simulink model "bianpinx1"  (R2015b)
settings: Solver=ode23t  StartTime=0.0  StopTime=0.4  RelTol=1e-3
libraries: powerlib x22, powerlib_extras x2
settings Model: Creator=Administrator  LastModifiedBy=Administrator
settings DataIOCC: SaveFormat=Array  SignalLoggingSaveFormat=ModelDataLogs
settings OptimizationCC: BooleanDataType=off  InitFltsAndDblsToZero=on
settings DebuggingCC: SaveWithParameterizedLinksMsg=none  UnderspecifiedInitializationDetection=Classic  MergeDetectMultiDrivingBlocksExec=none  SignalResolutionControl=TryResolveAllWithWarning  MaxConsecutiveZCsMsg=none  MultiTaskDSMMsg=warning  MultiTaskCondExecSysMsg=none  FcnCallInpInsideContextMsg=UseLocalSettings
settings HardwareCC: ProdBitPerPointer=32  ProdLargestAtomicFloat=None  ProdIntDivRoundTo=Undefined  ProdEndianess=Unspecified  ProdWordSize=32  ProdHWDeviceType=32-bit Generic  TargetUnknown=on
settings GRTTargetCC: TargetFcnLib=ansi_tfl_tmw.mat  CombineOutputUpdateFcns=off  GRTInterface=on
settings ConfigComp: CovModelRefEnable=Off

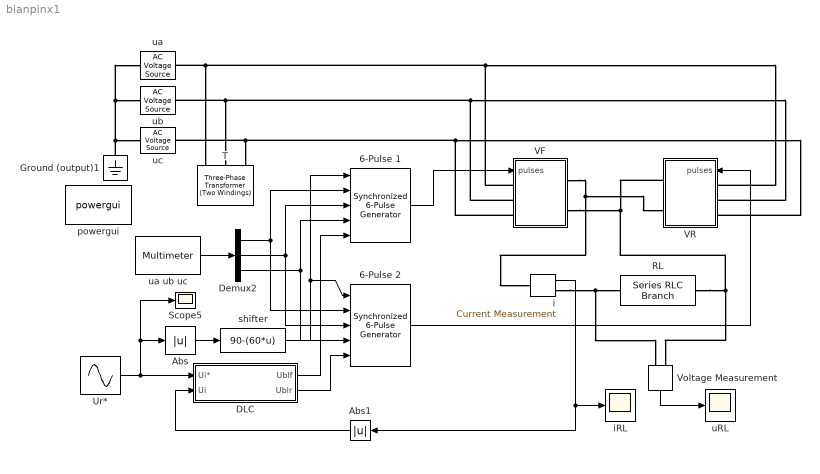
== system bianpinx1 ==
  "6-Pulse 1 " : powerlib_extras/Control  Blocks/Synchronized 6-Pulse Generator  freq=50  pwidth=10  Double_Pulse=on
  6-Pulse 2 : powerlib_extras/Control  Blocks/Synchronized 6-Pulse Generator  freq=50  pwidth=10  Double_Pulse=on
  Abs : Abs  SaturateOnIntegerOverflow=on
  Abs1 : Abs  SaturateOnIntegerOverflow=on
  DLC : Subsystem
  Demux2 : Demux  Outputs=3
  Ground (output)1 : powerlib/Elements/Ground  LConnTagsString=a
  RL : powerlib/Elements/Series RLC Branch  LConnTagsString=__new0  RConnTagsString=__new0  BranchType=RL  Resistance=1  Inductance=0.01  SetiL0=off  InitialCurrent=0  Capacitance=[]  Setx0=off  InitialVoltage=0  Measurements=Branch voltage and current
  Scope5 : Scope
  T : powerlib/Elements/Three-Phase Transformer (Two Windings)  Winding1Connection=Y  Winding2Connection=Y  CoreType=Three single-phase transformers  SetSaturation=off  Hysteresis=off  DataFile='basic_model'  SetInitialFlux=off  Measurements=Winding voltages  UNITS=pu  NominalPower=[ 250e6 , 50 ]  Winding1=[380, 0.002 , 0.08 ]  Winding2=[12.25 , 0.002 , 0.08 ]  Rm=500  Lm=500  L0=0.5  Saturation="[ 0,0  ;  0.005,1.2  ;  1.0,1.4 ]"  InitialFluxes=[ 0.8 , -0.8 , 0.7 ]  MoreParameters=off  BreakLoop=off  DataType=off  TransfoNumber=0
  Ur* : Sin  Frequency=2*pi*10  SampleTime=0
  VF : Subsystem  AncestorBlock=|  mask(Six-pulse thyristor bridge){Ron=0.01, Lon=10e-6, Rs=1e3, Cs=1e-6}
      | powerlib_extras/Three-Phase
      | Library/6 - pulse
      |  thyristor bridge
      mask prompts: Ron "Thyristor on-state resitance (Ohms) :"; Lon "Thyristor on-state inductance (H) :"; Rs "Snubber resistance (Ohms) :"; Cs "Snubber capacitance (F) :"
      mask help:
      | This block implements a six-pulses thyristor bridge rectifier with RC snubbers. Set the snubber resistance to Inf to remove all the thyristors snubbers. This block uses six Simplified Thyristors from the powerlib/Power Electronics library.
      | Input four (labeled 'pulses') of the block is a Simulink vector of length six that  controls the thyristors gates. Use the 'Look Under Mask' in the Edit menu  to see how the control vector operates the six thyrsistors.
      mask init:
      | power_initmask();
      settings: OpenFcn=power_openblockproxy()
      mask Display: plot(0,0,100,100,[50,50,35,50,65,50],[30,40,40,60,40,40],[35,65],[60,60],[50,50],[60,70],[45,40],[60,65],[35,40],[65,65])
  VR : Subsystem  AncestorBlock=|  mask(Six-pulse thyristor bridge){Ron=0.01, Lon=10e-6, Rs=1e3, Cs=1e-6}
      | powerlib_extras/Three-Phase
      | Library/6 - pulse
      |  thyristor bridge
      mask prompts: Ron "Thyristor on-state resitance (Ohms) :"; Lon "Thyristor on-state inductance (H) :"; Rs "Snubber resistance (Ohms) :"; Cs "Snubber capacitance (F) :"
      mask help:
      | This block implements a six-pulses thyristor bridge rectifier with RC snubbers. Set the snubber resistance to Inf to remove all the thyristors snubbers. This block uses six Simplified Thyristors from the powerlib/Power Electronics library.
      | Input four (labeled 'pulses') of the block is a Simulink vector of length six that  controls the thyristors gates. Use the 'Look Under Mask' in the Edit menu  to see how the control vector operates the six thyrsistors.
      mask init:
      | power_initmask();
      settings: OpenFcn=power_openblockproxy()
      mask Display: plot(0,0,100,100,[50,50,35,50,65,50],[30,40,40,60,40,40],[35,65],[60,60],[50,50],[60,70],[45,40],[60,65],[35,40],[65,65])
  Voltage Measurement : powerlib/Measurements/Voltage Measurement  PhasorSimulation=off  OutputType=Complex  PSBequivalent=0
  i : powerlib/Measurements/Current Measurement  PhasorSimulation=off  OutputType=Magnitude  PSBequivalent=0
  iRL : Scope
  powergui : powerlib/powergui  Priority=1  SimulationMode=Continuous  SolverType=Tustin/Backward Euler (TBE)  SampleTime=50e-6  frequency=60  SPID=off  DisableSnubberDevices=off  DisableRonSwitches=off  DisableVfSwitches=off  SwTol=0  DisplayEquations=off  Interpol=off  ExternalGateDelay=off  methode=off  Ts=10  FunctionMessages=off  echomessages=off  HookPort=off  EnableUseOfTLC=off  x0status=blocks  frequencyindice=50  Pbase=100e6  ErrMax=1e-4  Iterations=50  UnitsV=kV  UnitsW=MW  buscounter=0  RestoreLinks=warning  ResistiveCurrentMeasurement=off  Frange=[0:2:500]  Ylog=off  Xlog=on  ShowGrid=off  save=off  variable=ZData  structure=0  ZoomFFT=off  StartTime=0.0  cycles=1  DisplayStyle=1  fundamental=60  FreqAxis=off  MaxFrequency=1000  frequencyindicesteady=1  RmsSteady=1  display=off
  shifter : Fcn  Expr=90-(60*u)
  uRL : Scope
  ua : powerlib/Electrical Sources/AC Voltage Source  Amplitude=311  Phase=0  Frequency=50  SampleTime=0  Measurements=Voltage  BusType=swing  Pref=10e3  Qref=0  Qmin=-inf  Qmax=+inf
  ua ub uc : powerlib/Measurements/Multimeter  PhasorSimulation=off  OutputType=Magnitude  sel=[5 6 7]  L=11  Gain=[1 1 1]  yselected={'Uan_w2: T','Ubn_w2: T','Ucn_w2: T'};  PSBOutputType=1  PSBequivalent=0  AxesSetting=[0,0.1,-100,100]  Display=0  SavedBlockNames=-11
  ub : powerlib/Electrical Sources/AC Voltage Source  Amplitude=311  Phase=-120  Frequency=50  SampleTime=0  Measurements=Voltage  BusType=swing  Pref=10e3  Qref=0  Qmin=-inf  Qmax=+inf
  uc : powerlib/Electrical Sources/AC Voltage Source  Amplitude=311  Phase=-240  Frequency=50  SampleTime=0  Measurements=Voltage  BusType=swing  Pref=10e3  Qref=0  Qmin=-inf  Qmax=+inf
  wires:
  6-Pulse 2/1 -> VR/1(pulses)
  Ur*/1 -> Abs/1, Scope5/1, DLC/1(Ui*)
  DLC/1(Ublf) -> "6-Pulse 1 "/5
  DLC/2(Ublr) -> 6-Pulse 2/5
  Abs/1 -> shifter/1
  shifter/1 -> "6-Pulse 1 "/1, 6-Pulse 2/1
  Demux2/1 -> "6-Pulse 1 "/2, 6-Pulse 2/2
  Demux2/2 -> "6-Pulse 1 "/3, 6-Pulse 2/3
  Demux2/3 -> "6-Pulse 1 "/4, 6-Pulse 2/4
  Abs1/1 -> DLC/2(Ui)
  ua ub uc/1 -> Demux2/1
  i/1 -> Abs1/1, iRL/1
  Voltage Measurement/1 -> uRL/1
  "6-Pulse 1 "/1 -> VF/1(pulses)
  connections:
  Ground (output)1/LConn1 -- ua/LConn1 -- ub/LConn1 -- uc/LConn1
  i/RConn1 -- RL/LConn1 -- Voltage Measurement/LConn1
  RL/RConn1 -- VF/RConn2 -- VR/RConn1 -- Voltage Measurement/LConn2
  VF/RConn1 -- VR/RConn2 -- i/LConn1
  VF/LConn1 -- VR/LConn1 -- ua/RConn1 -- T/LConn1
  VF/LConn2 -- VR/LConn2 -- ub/RConn1 -- T/LConn2
  VF/LConn3 -- VR/LConn3 -- uc/RConn1 -- T/LConn3

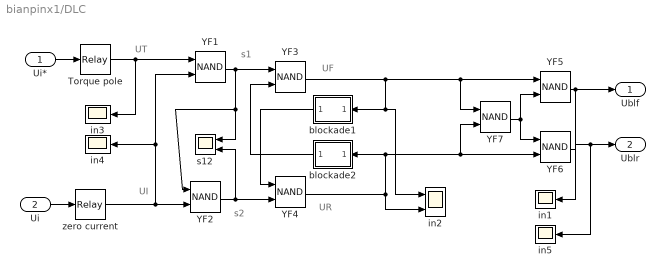
== system bianpinx1/DLC ==
  note: s1
  note: s2
  note: UT
  note: UI
  note: UF
  note: UR
  Ui* : Inport
  Ui : Inport  Port=2
  Torque pole : Relay  OnSwitchValue=0.001  OffSwitchValue=-0.001
  YF{1..7} (7 alike) : Logic  Operator=NAND
  blockade1 : Subsystem
  blockade2 : Subsystem
  in{1,3..5} (4 alike) : Scope
  in2 : Scope  NumInputPorts=2
  s12 : Scope  NumInputPorts=2
  "zero current  " : Relay  OnSwitchValue=0.5  OffSwitchValue=0.01  OnOutputValue=0  OffOutputValue=1
  Ublf : Outport
  Ublr : Outport  Port=2
  wires:
  YF1/1 -> YF3/1, YF2/1, s12/1
  YF2/1 -> YF4/2, s12/2
  YF4/1 -> in2/2, YF7/2, YF6/2, blockade2/1(In1)
  "zero current  "/1 -> YF2/2, YF1/2, in4/1
  YF3/1 -> YF7/1, YF5/1, in2/1, blockade1/1(In1)
  YF7/1 -> YF5/2, YF6/1
  Torque pole/1 -> YF1/1, in3/1
  Ui*/1 -> Torque pole/1
  YF5/1 -> Ublf/1, in1/1
  YF6/1 -> Ublr/1, in5/1
  Ui/1 -> "zero current  "/1
  blockade1/1(Out1) -> YF4/1
  blockade2/1(Out1) -> YF3/2

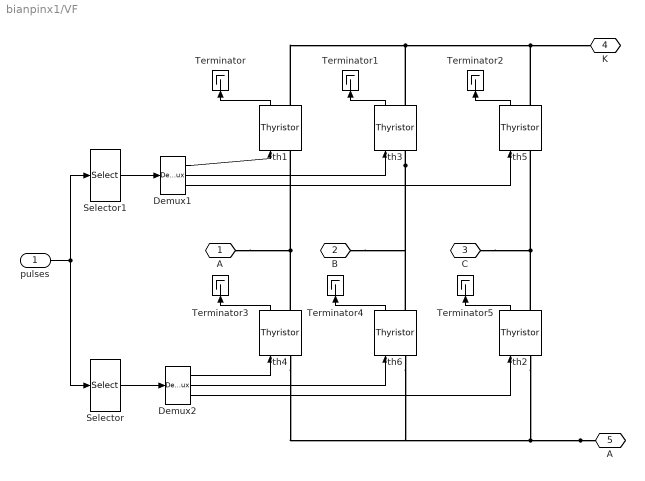
== system bianpinx1/VF ==
  pulses : Inport
  Demux1 : Demux  Outputs=3
  Demux2 : Demux  Outputs=3
  Selector : Selector  InputPortWidth=6  IndexOptions=Index vector (dialog)  Indices=[ 4 6 2]  OutputSizes=1
  Selector1 : Selector  InputPortWidth=6  IndexOptions=Index vector (dialog)  Indices=[ 1 3 5]  OutputSizes=1
  Terminator{,1..5} (6 alike) : Terminator
  th{1..6} (6 alike) : powerlib/Power Electronics/Thyristor  Ron=Ron  Lon=Lon  Vf=0  IC=0  Rs=Rs  Cs=Cs  Measurements=on
  A : PMIOPort  Port=1  Side=Left
  B : PMIOPort  Port=2  Side=Left
  C : PMIOPort  Port=3  Side=Left
  "K " : PMIOPort  Port=4  Side=Right
  "A " : PMIOPort  Port=5  Side=Right
  wires:
  Selector/1 -> Demux2/1
  Selector1/1 -> Demux1/1
  pulses/1 -> Selector1/1, Selector/1
  th1/1 -> Terminator/1
  th3/1 -> Terminator1/1
  th5/1 -> Terminator2/1
  th2/1 -> Terminator5/1
  th6/1 -> Terminator4/1
  th4/1 -> Terminator3/1
  Demux1/1 -> th1/1
  Demux1/2 -> th3/1
  Demux1/3 -> th5/1
  Demux2/1 -> th4/1
  Demux2/2 -> th6/1
  Demux2/3 -> th2/1
  connections:
  th3/RConn1 -- th1/RConn1 -- "K "/RConn1 -- th5/RConn1
  A/RConn1 -- th4/RConn1 -- th1/LConn1
  th3/LConn1 -- th6/RConn1 -- B/RConn1
  C/RConn1 -- th2/RConn1 -- th5/LConn1
  "A "/RConn1 -- th6/LConn1 -- th4/LConn1 -- th2/LConn1

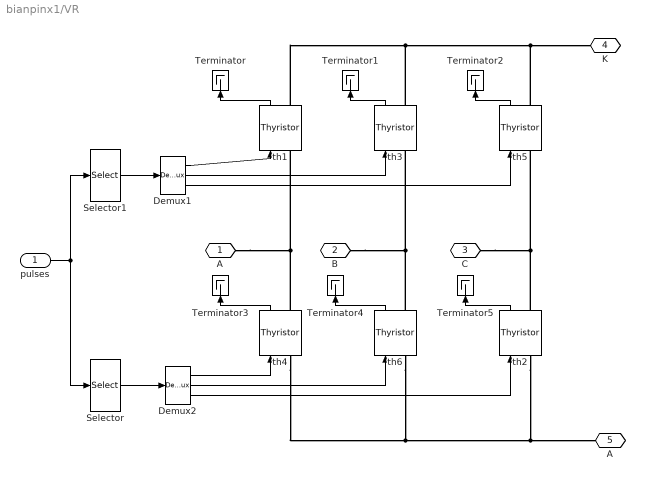
== system bianpinx1/VR ==
  pulses : Inport
  Demux1 : Demux  Outputs=3
  Demux2 : Demux  Outputs=3
  Selector : Selector  InputPortWidth=6  IndexOptions=Index vector (dialog)  Indices=[ 4 6 2]  OutputSizes=1
  Selector1 : Selector  InputPortWidth=6  IndexOptions=Index vector (dialog)  Indices=[ 1 3 5]  OutputSizes=1
  Terminator{,1..5} (6 alike) : Terminator
  th{1..6} (6 alike) : powerlib/Power Electronics/Thyristor  Ron=Ron  Lon=Lon  Vf=0  IC=0  Rs=Rs  Cs=Cs  Measurements=on
  A : PMIOPort  Port=1  Side=Left
  B : PMIOPort  Port=2  Side=Left
  C : PMIOPort  Port=3  Side=Left
  "K " : PMIOPort  Port=4  Side=Right
  "A " : PMIOPort  Port=5  Side=Right
  wires:
  Selector/1 -> Demux2/1
  Selector1/1 -> Demux1/1
  pulses/1 -> Selector1/1, Selector/1
  th1/1 -> Terminator/1
  th3/1 -> Terminator1/1
  th5/1 -> Terminator2/1
  th2/1 -> Terminator5/1
  th6/1 -> Terminator4/1
  th4/1 -> Terminator3/1
  Demux1/1 -> th1/1
  Demux1/2 -> th3/1
  Demux1/3 -> th5/1
  Demux2/1 -> th4/1
  Demux2/2 -> th6/1
  Demux2/3 -> th2/1
  connections:
  th1/RConn1 -- th3/RConn1 -- th5/RConn1 -- "K "/RConn1
  th4/RConn1 -- th1/LConn1 -- A/RConn1
  th6/RConn1 -- B/RConn1 -- th3/LConn1
  th2/RConn1 -- th5/LConn1 -- C/RConn1
  th4/LConn1 -- th2/LConn1 -- "A "/RConn1 -- th6/LConn1

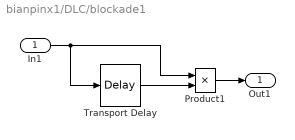
== system bianpinx1/DLC/blockade1 ==
  In1 : Inport
  Product1 : Product  SaturateOnIntegerOverflow=on  RndMeth=Zero  InputSameDT=on  OutDataTypeStr=Inherit: Same as first input
  Transport Delay : TransportDelay  DelayTime=0.001
  Out1 : Outport
  wires:
  In1/1 -> Product1/1, Transport Delay/1
  Transport Delay/1 -> Product1/2
  Product1/1 -> Out1/1

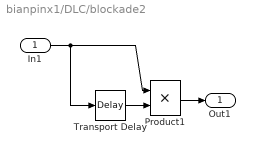
== system bianpinx1/DLC/blockade2 ==
  In1 : Inport
  Product1 : Product  SaturateOnIntegerOverflow=on  RndMeth=Zero  InputSameDT=on  OutDataTypeStr=Inherit: Same as first input
  Transport Delay : TransportDelay  DelayTime=0.001
  Out1 : Outport
  wires:
  Product1/1 -> Out1/1
  Transport Delay/1 -> Product1/2
  In1/1 -> Transport Delay/1, Product1/1
